simulink model "untitled"  (R2016a)
settings: Solver=VariableStepAuto  StartTime=0.0  StopTime=50  RelTol=1e-3
settings Model: Creator=Elias-k  LastModifiedBy=Elias-k

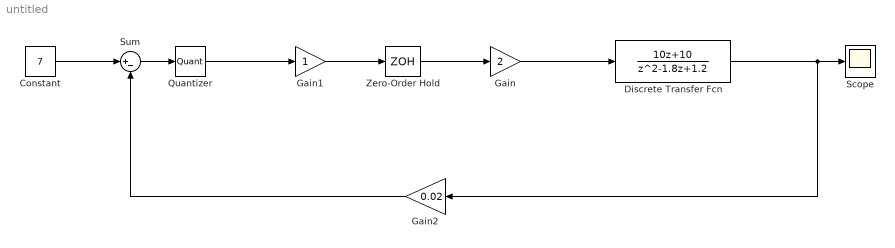
== system untitled ==
  Constant : Constant  Value=7
  Discrete Transfer Fcn : DiscreteTransferFcn  Numerator=[10 10]  Denominator=[1 -1.8 1.2]  SampleTime=1
  Gain : Gain  Gain=2
  Gain1 : Gain
  Gain2 : Gain  Gain=0.02
  Quantizer : Quantizer  QuantizationInterval=0.0390625
  Scope : Scope
  Sum : Sum  Inputs=|+-
  Zero-Order Hold : ZeroOrderHold
  wires:
  Quantizer/1 -> Gain1/1
  Gain/1 -> Discrete Transfer Fcn/1
  Discrete Transfer Fcn/1 -> Gain2/1, Scope/1
  Zero-Order Hold/1 -> Gain/1
  Gain1/1 -> Zero-Order Hold/1
  Sum/1 -> Quantizer/1
  Constant/1 -> Sum/1
  Gain2/1 -> Sum/2
